simulink model "modele_complet_simulink2024"  (R2024a)
settings: Solver=VariableStepAuto  StartTime=0.0  StopTime=T_att  RelTol=1e-3
values from neighbouring files (symbols this model uses):
  d = 4    [script_devoir2.m]
  g = 9.81    [script_devoir2.m]
  isQ3a = false    [script_devoir2.m]
  J = 6000    [script_devoir2.m]
  Kdtheta = 13.4    [script_devoir2.m]
  Kdx = -0.367    [script_devoir2.m]
  Kdy = 15000    [script_devoir2.m]
  Kitheta = 0.6    [script_devoir2.m]
  Kix = -0.176    [script_devoir2.m]
  Kiy = 125000    [script_devoir2.m]
  Kptheta = 39.5    [script_devoir2.m]
  Kpx = -0.440    (= -0.44)    [script_devoir2.m]
  Kpy = 75000    [script_devoir2.m]
  m = 1000    [script_devoir2.m]
  x0 = [x0_pos; vx0; y0_pos; vy0; 0; 0]    [script_devoir2.m]
settings Model: Creator=Andrea  LastModifiedBy=Andrea
settings ConfigComp: CovBoundaryAbsTol=1.0e-5

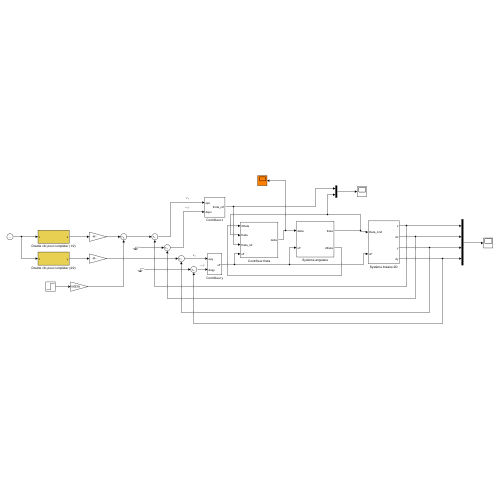
[thumbnail: Simulink's stored preview of the top-level diagram]
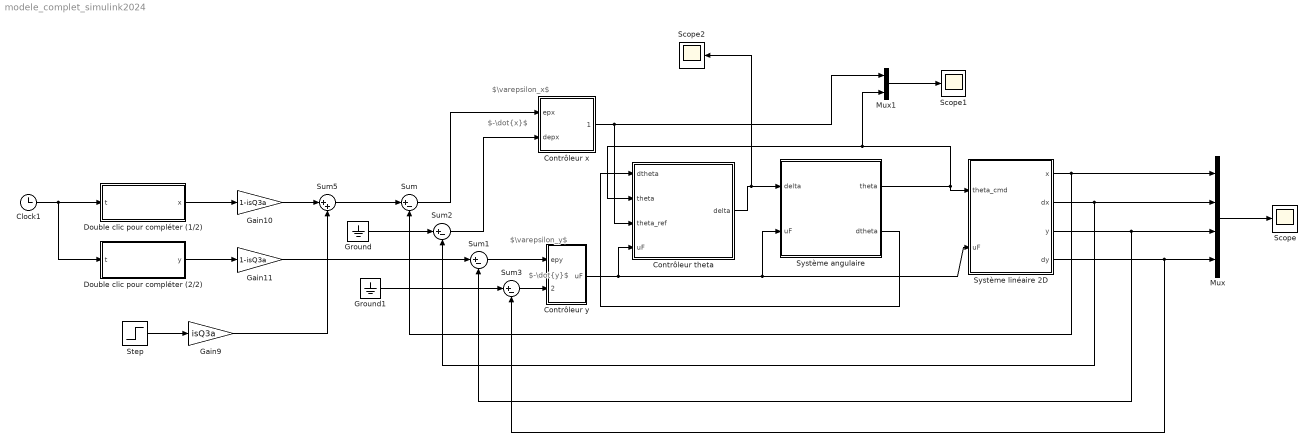
== system modele_complet_simulink2024 ==
  note: $\varepsilon_x$
  note: $-\dot{y}$
  note: $-\dot{x}$
  note: $\varepsilon_y$
  Clock1 : Clock
  Contrôleur theta : Subsystem
  Contrôleur x : Subsystem
  Contrôleur y : Subsystem
  Double clic pour compléter (1/2) : Subsystem
  Double clic pour compléter (2/2) : Subsystem
  Gain10 : Gain  Gain=1-isQ3a
  Gain11 : Gain  Gain=1-isQ3a
  Gain9 : Gain  Gain=isQ3a
  Ground : Ground
  Ground1 : Ground
  Mux : Mux
  Mux1 : Mux  Inputs=2
  Scope : Scope
  Scope1 : Scope
  Scope2 : Scope
  Step : Step  Time=0  SampleTime=0
  Sum{,1..3} (4 alike) : Sum  Inputs=|+-
  Sum5 : Sum  Inputs=|++
  Système angulaire : Subsystem
  Système linéaire 2D : Subsystem
  wires:
  Sum2/1 -> Contrôleur x/2(depx)
  Système linéaire 2D/3(y) -> Sum1/2, Mux/3
  Système linéaire 2D/1(x) -> Sum/2, Mux/1
  Contrôleur x/1(theta_ref) -> Mux1/1, Contrôleur theta/3(theta_ref)
  Système linéaire 2D/2(dx) -> Sum2/2, Mux/2
  Sum/1 -> Contrôleur x/1(epx)
  Système linéaire 2D/4(dy) -> Sum3/2, Mux/4
  Mux/1 -> Scope/1
  Ground/1 -> Sum2/1
  Ground1/1 -> Sum3/1
  Mux1/1 -> Scope1/1
  Contrôleur theta/1(delta) -> Système angulaire/1(delta), Scope2/1
  Système angulaire/1(theta) -> Mux1/2, Contrôleur theta/2(theta), Système linéaire 2D/1(theta_cmd)
  Système angulaire/2(dtheta) -> Contrôleur theta/1(dtheta)
  Sum1/1 -> Contrôleur y/1(epy)
  Sum3/1 -> Contrôleur y/2(depy)
  Double clic pour compléter (2/2)/1(y) -> Gain11/1
  Gain9/1 -> Sum5/2
  Step/1 -> Gain9/1
  Clock1/1 -> Double clic pour compléter (1/2)/1(t), Double clic pour compléter (2/2)/1(t)
  Double clic pour compléter (1/2)/1(x) -> Gain10/1
  Gain10/1 -> Sum5/1
  Sum5/1 -> Sum/1
  Gain11/1 -> Sum1/1
  Contrôleur y/1(uF) -> Système angulaire/2(uF), Système linéaire 2D/2(uF), Contrôleur theta/4(uF)

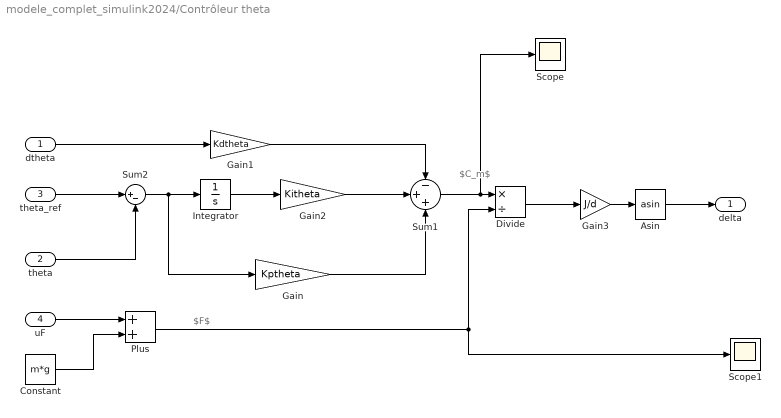
== system modele_complet_simulink2024/Contrôleur theta ==
  note: $F$
  note: $C_m$
  dtheta : Inport
  theta : Inport  Port=2
  theta_ref : Inport  Port=3
  uF : Inport  Port=4
  Asin : Trigonometry  Operator=asin
  Constant : Constant  Value=m*g
  Divide : Product  Inputs=*/
  Gain : Gain  Gain=Kptheta
  Gain1 : Gain  Gain=Kdtheta
  Gain2 : Gain  Gain=Kitheta
  Gain3 : Gain  Gain=J/d
  Integrator : Integrator
  Plus : Sum
  Scope : Scope
  Scope1 : Scope
  Sum1 : Sum  Inputs=-++
  Sum2 : Sum  Inputs=|+-
  delta : Outport
  wires:
  Gain1/1 -> Sum1/1
  Gain/1 -> Sum1/3
  dtheta/1 -> Gain1/1
  Asin/1 -> delta/1
  Divide/1 -> Gain3/1
  Gain2/1 -> Sum1/2
  theta_ref/1 -> Sum2/1
  Sum1/1 -> Scope/1, Divide/1
  Gain3/1 -> Asin/1
  Sum2/1 -> Gain/1, Integrator/1
  theta/1 -> Sum2/2
  uF/1 -> Plus/1
  Constant/1 -> Plus/2
  Integrator/1 -> Gain2/1
  Plus/1 -> Scope1/1, Divide/2

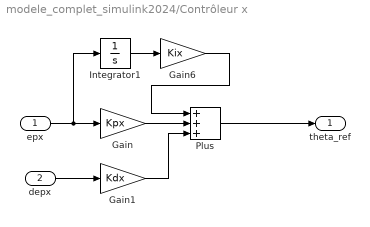
== system modele_complet_simulink2024/Contrôleur x ==
  epx : Inport
  depx : Inport  Port=2
  Gain : Gain  Gain=Kpx
  Gain1 : Gain  Gain=Kdx
  Gain6 : Gain  Gain=Kix
  Integrator1 : Integrator
  Plus : Sum  Inputs=+++
  theta_ref : Outport
  wires:
  Integrator1/1 -> Gain6/1
  epx/1 -> Integrator1/1, Gain/1
  depx/1 -> Gain1/1
  Gain1/1 -> Plus/3
  Gain6/1 -> Plus/1
  Gain/1 -> Plus/2
  Plus/1 -> theta_ref/1

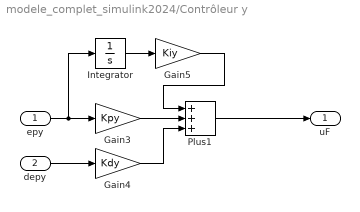
== system modele_complet_simulink2024/Contrôleur y ==
  epy : Inport
  depy : Inport  Port=2
  Gain3 : Gain  Gain=Kpy
  Gain4 : Gain  Gain=Kdy
  Gain5 : Gain  Gain=Kiy
  Integrator : Integrator
  Plus1 : Sum  Inputs=+++
  uF : Outport
  wires:
  Gain3/1 -> Plus1/2
  Plus1/1 -> uF/1
  depy/1 -> Gain4/1
  Integrator/1 -> Gain5/1
  Gain4/1 -> Plus1/3
  Gain5/1 -> Plus1/1
  epy/1 -> Integrator/1, Gain3/1

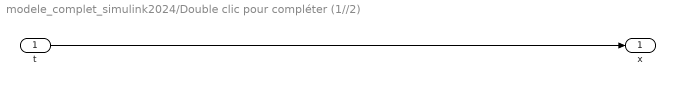
== system modele_complet_simulink2024/Double clic pour compléter (1//2) ==
  t : Inport
  x : Outport
  wires:
  t/1 -> x/1

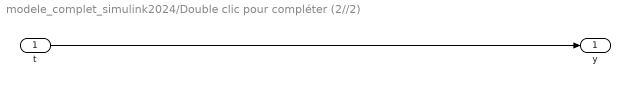
== system modele_complet_simulink2024/Double clic pour compléter (2//2) ==
  t : Inport
  y : Outport
  wires:
  t/1 -> y/1

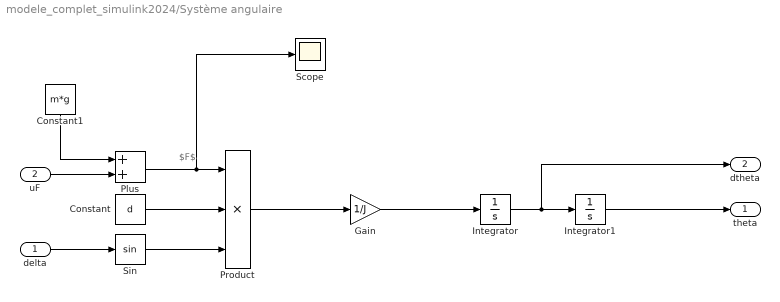
== system modele_complet_simulink2024/Système angulaire ==
  note: $F$
  delta : Inport
  uF : Inport  Port=2
  Constant : Constant  Value=d
  Constant1 : Constant  Value=m*g
  Gain : Gain  Gain=1/J
  Integrator : Integrator
  Integrator1 : Integrator
  Plus : Sum
  Product : Product  Inputs=3
  Scope : Scope
  Sin : Trigonometry
  theta : Outport
  dtheta : Outport  Port=2
  wires:
  Integrator/1 -> dtheta/1, Integrator1/1
  Gain/1 -> Integrator/1
  Integrator1/1 -> theta/1
  Product/1 -> Gain/1
  Constant/1 -> Product/2
  delta/1 -> Sin/1
  Sin/1 -> Product/3
  Plus/1 -> Scope/1, Product/1
  uF/1 -> Plus/2
  Constant1/1 -> Plus/1

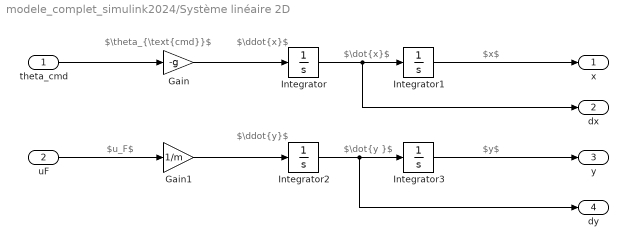
== system modele_complet_simulink2024/Système linéaire 2D ==
  note: $\ddot{y}$
  note: $u_F$
  note: $\theta_{\text{cmd}}$
  note: $x$
  note: $\dot{x}$
  note: $\ddot{x}$
  note: $\dot{y }$
  note: $y$
  theta_cmd : Inport
  uF : Inport  Port=2
  Gain : Gain  Gain=-g
  Gain1 : Gain  Gain=1/m
  Integrator : Integrator  InitialCondition=x0(2)
  Integrator1 : Integrator  InitialCondition=x0(1)
  Integrator2 : Integrator  InitialCondition=x0(4)
  Integrator3 : Integrator  InitialCondition=x0(3)
  x : Outport
  dx : Outport  Port=2
  y : Outport  Port=3
  dy : Outport  Port=4
  wires:
  Gain1/1 -> Integrator2/1
  theta_cmd/1 -> Gain/1
  Integrator3/1 -> y/1
  Integrator/1 -> dx/1, Integrator1/1
  Gain/1 -> Integrator/1
  Integrator1/1 -> x/1
  Integrator2/1 -> dy/1, Integrator3/1
  uF/1 -> Gain1/1
